simulink model "modelo"  (R2013a)
settings: Solver=ode45  StartTime=0.0  StopTime=50  FixedStep=0.01  RelTol=1e-3
values from neighbouring files (symbols this model uses):
  Hmax = [10 12 11 9]    [ini.m]
  Itot = [Ixx Ixy Izx; Ixy Iyy Iyz; Izx Iyz Izz]    [ini.m]
  Itot_inv = inv(Itot)    [ini.m]
  Iws = [5 5 5 5]    [ini.m]
  omega0 = [2000 2000 2000 2000]*rpm2r    [ini.m]
  r2d = 180/pi    (= 57.2957795131)    [ini.m]
  tau = [10;0;0]    [ini.m]
  w0 = [0.2 0.15 -0.18]*(pi/180.0)    [ini.m]
  w1 = [-1 -1 -1]/sqrt(3)    [ini.m]
  w2 = [-1 -1 +1]/sqrt(3)    [ini.m]
  w3 = [-1 +1 +1]/sqrt(3)    [ini.m]
  w4 = [-1 +1 -1]/sqrt(3)    [ini.m]
settings Model: Creator=henry  LastModifiedBy=henry
settings DataIOCC: InspectSignalLogs=on

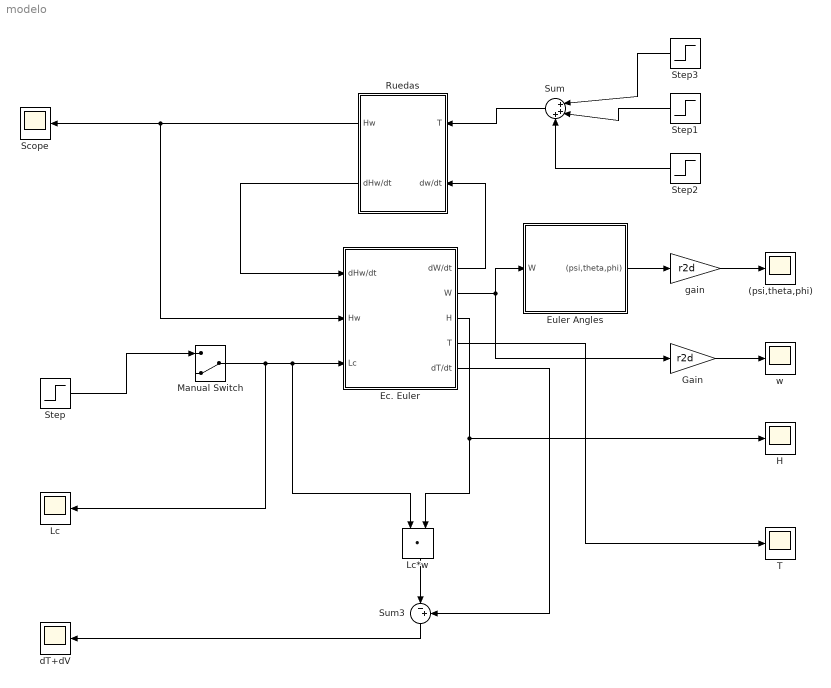
== system modelo ==
  (psi,theta,phi) : Scope
      settings: TickLabels=on  ShowLegends=on
  Ec. Euler : Subsystem
  Euler Angles : Subsystem
  Gain : Gain  Gain=r2d
  H : Scope
      settings: ShowLegends=on  SaveName=ScopeData4
  Lc : Scope
      settings: TickLabels=on  ShowLegends=on  SaveName=ScopeData2
  Lc*w : DotProduct  InputSameDT=on  OutDataTypeStr=Inherit: Inherit via internal rule
  Manual Switch : ManualSwitch  CurrentSetting=0
  Ruedas : Subsystem
  Scope : Scope
      settings: ShowLegends=on  SaveName=ScopeData9
  Step : Step  Time=1000  Before=[0;0;0]  After=tau  SampleTime=0
  Step1 : Step  Time=0  Before=[0;0;0]  After=tau  SampleTime=0
  Step2 : Step  Time=10  Before=[0;0;0]  After=-2*tau  SampleTime=0
  Step3 : Step  Time=15  Before=[0;0;0]  After=tau  SampleTime=0
  Sum : Sum  Inputs=|+++
  Sum3 : Sum  Inputs=|-+
  T : Scope
      settings: SaveName=ScopeData6
  dT+dV : Scope
      settings: TickLabels=on  ShowLegends=on  SaveName=ScopeData5
  gain : Gain  Gain=r2d
  w : Scope
      settings: TickLabels=on  ShowLegends=on
  wires:
  Lc*w/1 -> Sum3/1
  Sum3/1 -> dT+dV/1
  Ec. Euler/4(T) -> T/1
  Ec. Euler/5(dT/dt) -> Sum3/2
  Euler Angles/1((psi,theta,phi)) -> gain/1
  Gain/1 -> w/1
  gain/1 -> (psi,theta,phi)/1
  Ec. Euler/3(H) -> Lc*w/2, H/1
  Ec. Euler/2(W) -> Gain/1, Euler Angles/1(W)
  Ec. Euler/1(dW/dt) -> Ruedas/2(dw/dt)
  Ruedas/1(Hw) -> Ec. Euler/2(Hw), Scope/1
  Ruedas/2(dHw/dt) -> Ec. Euler/1(dHw/dt)
  Step1/1 -> Sum/2
  Step/1 -> Manual Switch/1
  Manual Switch/1 -> Lc/1, Lc*w/1, Ec. Euler/3(Lc)
  Step2/1 -> Sum/3
  Sum/1 -> Ruedas/1(T)
  Step3/1 -> Sum/1

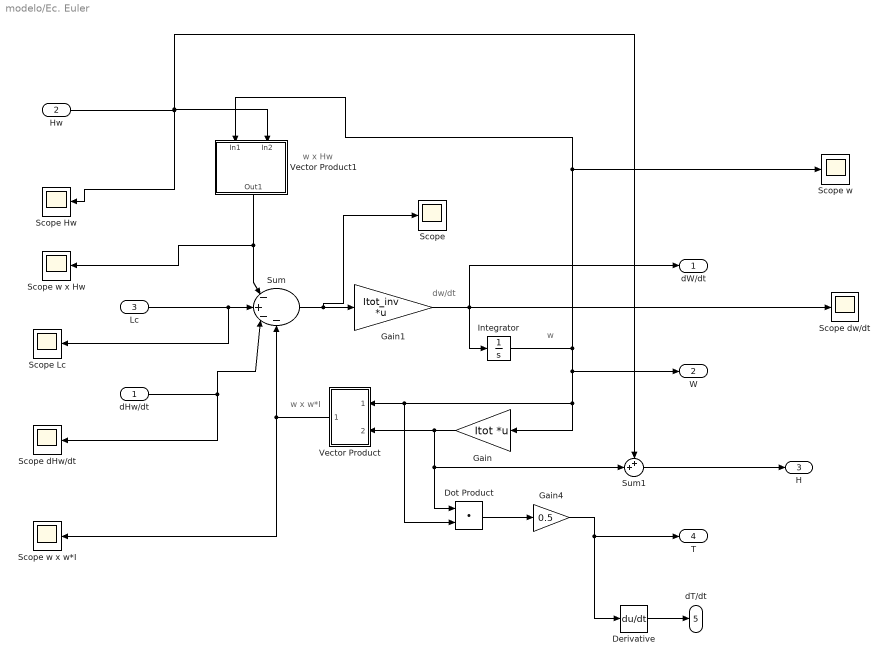
== system modelo/Ec. Euler ==
  note: w x w*I
  note: w x Hw
  note: w
  note: dw/dt
  dHw/dt : Inport
  Hw : Inport  Port=2
  Lc : Inport  Port=3
  Derivative : Derivative
  Dot Product : DotProduct  InputSameDT=on  OutDataTypeStr=Inherit: Inherit via internal rule
  Gain : Gain  Gain=Itot  Multiplication=Matrix(K*u)
  Gain1 : Gain  Gain=Itot_inv  Multiplication=Matrix(K*u)
  Gain4 : Gain  Gain=0.5
  Integrator : Integrator  InitialCondition=w0
  Scope : Scope
      settings: SaveName=ScopeData11
  Scope Hw : Scope
      settings: SaveName=ScopeData17
  Scope Lc : Scope
      settings: SaveName=ScopeData13
  Scope dHw/dt : Scope
      settings: SaveName=ScopeData14
  Scope dw/dt : Scope
      settings: SaveName=ScopeData18
  Scope w : Scope
      settings: SaveName=ScopeData16
  Scope w x Hw : Scope
      settings: SaveName=ScopeData15
  Scope w x w*I : Scope
      settings: SaveName=ScopeData19
  Sum : Sum  Inputs=|-+--
  Sum1 : Sum  Inputs=++|
  Vector Product : Subsystem
  Vector Product1 : Subsystem
  dW/dt : Outport
  W : Outport  Port=2
  H : Outport  Port=3
  T : Outport  Port=4
  dT/dt : Outport  Port=5
  wires:
  Vector Product/1(Out1) -> Scope w x w*I/1, Sum/4
  Gain/1 -> Sum1/2, Dot Product/1, Vector Product/2(In2)
  Gain1/1 -> dW/dt/1, Scope dw/dt/1, Integrator/1
  Derivative/1 -> dT/dt/1
  Integrator/1 -> W/1, Dot Product/2, Vector Product/1(In1), Gain/1, Vector Product1/1(In1), Scope w/1
  Lc/1 -> Scope Lc/1, Sum/2
  Dot Product/1 -> Gain4/1
  Gain4/1 -> T/1, Derivative/1
  dHw/dt/1 -> Sum/3, Scope dHw/dt/1
  Vector Product1/1(Out1) -> Sum/1, Scope w x Hw/1
  Hw/1 -> Scope Hw/1, Vector Product1/2(In2), Sum1/1
  Sum/1 -> Scope/1, Gain1/1
  Sum1/1 -> H/1

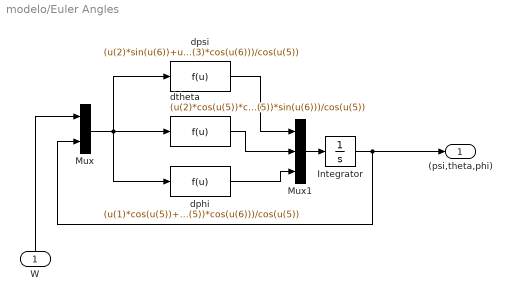
== system modelo/Euler Angles ==
  W : Inport
  Integrator : Integrator
  Mux : Mux  Inputs=2
  Mux1 : Mux  Inputs=3
  dphi : Fcn  Expr=(u(1)*cos(u(5))+u(2)*sin(u(5))*sin(u(6))+u(3)*sin(u(5))*cos(u(6)))/cos(u(5))
  dpsi : Fcn  Expr=(u(2)*sin(u(6))+u(3)*cos(u(6)))/cos(u(5))
  dtheta : Fcn  Expr=(u(2)*cos(u(5))*cos(u(6))-u(3)*cos(u(5))*sin(u(6)))/cos(u(5))
  (psi,theta,phi) : Outport
  wires:
  Integrator/1 -> (psi,theta,phi)/1, Mux/2
  dphi/1 -> Mux1/3
  dtheta/1 -> Mux1/2
  Mux1/1 -> Integrator/1
  dpsi/1 -> Mux1/1
  Mux/1 -> dpsi/1, dphi/1, dtheta/1
  W/1 -> Mux/1

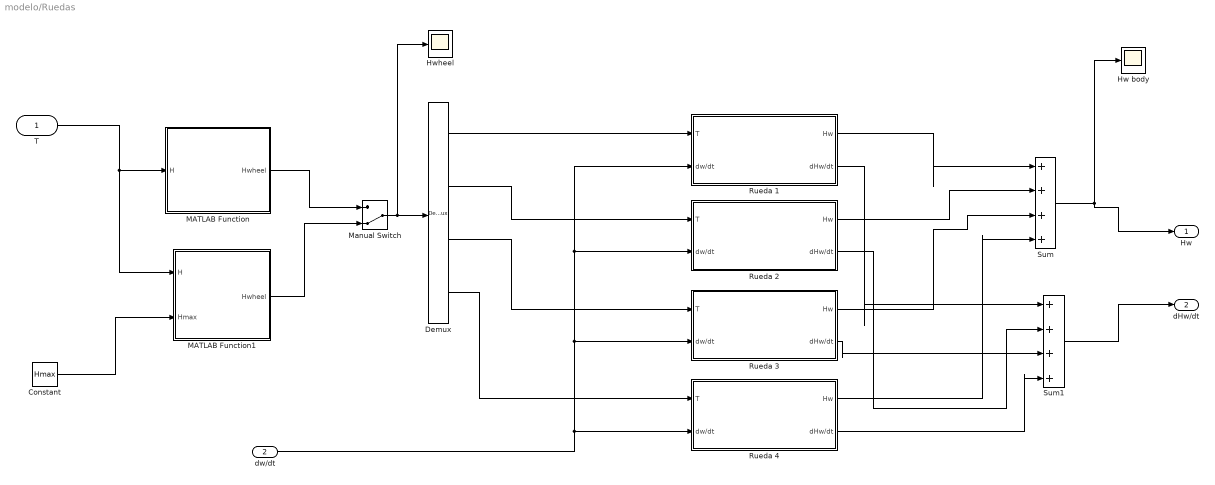
== system modelo/Ruedas ==
  T : Inport
  dw/dt : Inport  Port=2
  Constant : Constant  Value=Hmax
  Demux : Demux
  Hw body : Scope
      settings: ShowLegends=on  SaveName=ScopeData7
  Hwheel : Scope
      settings: ShowLegends=on  SaveName=ScopeData8
  MATLAB Function : MATLAB Function  TreatAsAtomicUnit=on
  MATLAB Function1 : MATLAB Function  TreatAsAtomicUnit=on
  Manual Switch : ManualSwitch  CurrentSetting=0
  Rueda 1 : Subsystem
  Rueda 2 : Subsystem
  Rueda 3 : Subsystem
  Rueda 4 : Subsystem
  Sum : Sum  Inputs=|++++
  Sum1 : Sum  Inputs=|++++
  Hw : Outport
  dHw/dt : Outport  Port=2
  wires:
  T/1 -> MATLAB Function1/1(H), MATLAB Function/1(H)
  Demux/1 -> Rueda 1/1(T)
  dw/dt/1 -> Rueda 2/2(dw/dt), Rueda 1/2(dw/dt), Rueda 3/2(dw/dt), Rueda 4/2(dw/dt)
  Demux/2 -> Rueda 2/1(T)
  Demux/3 -> Rueda 3/1(T)
  Demux/4 -> Rueda 4/1(T)
  Rueda 1/1(Hw) -> Sum/1
  Rueda 2/1(Hw) -> Sum/2
  Rueda 3/1(Hw) -> Sum/3
  Rueda 4/1(Hw) -> Sum/4
  Rueda 1/2(dHw/dt) -> Sum1/1
  Rueda 2/2(dHw/dt) -> Sum1/2
  Rueda 3/2(dHw/dt) -> Sum1/3
  Rueda 4/2(dHw/dt) -> Sum1/4
  Sum1/1 -> dHw/dt/1
  Sum/1 -> Hw/1, Hw body/1
  Constant/1 -> MATLAB Function1/2(Hmax)
  MATLAB Function1/1(Hwheel) -> Manual Switch/2
  MATLAB Function/1(Hwheel) -> Manual Switch/1
  Manual Switch/1 -> Hwheel/1, Demux/1

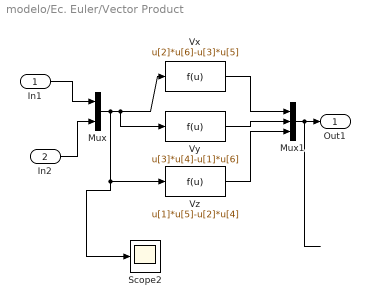
== system modelo/Ec. Euler/Vector Product ==
  In1 : Inport
  In2 : Inport  Port=2
  Mux : Mux  Inputs=2
  Mux1 : Mux  Inputs=3
  Scope2 : Scope
      settings: ShowLegends=on  SaveName=ScopeData3
  Vx : Fcn  Expr=u[2]*u[6]-u[3]*u[5]
  Vy : Fcn  Expr=u[3]*u[4]-u[1]*u[6]
  Vz : Fcn  Expr=u[1]*u[5]-u[2]*u[4]
  Out1 : Outport
  wires:
  In2/1 -> Mux/2
  Mux1/1 -> Out1/1
  In1/1 -> Mux/1
  Vz/1 -> Mux1/3
  Vy/1 -> Mux1/2
  Vx/1 -> Mux1/1
  Mux/1 -> Vz/1, Scope2/1, Vy/1, Vx/1

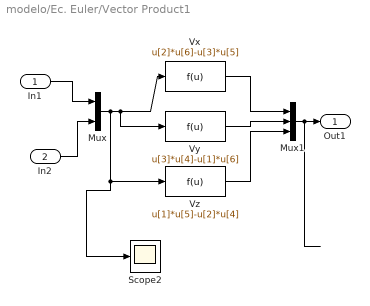
== system modelo/Ec. Euler/Vector Product1 ==
  In1 : Inport
  In2 : Inport  Port=2
  Mux : Mux  Inputs=2
  Mux1 : Mux  Inputs=3
  Scope2 : Scope
      settings: ShowLegends=on  SaveName=ScopeData3
  Vx : Fcn  Expr=u[2]*u[6]-u[3]*u[5]
  Vy : Fcn  Expr=u[3]*u[4]-u[1]*u[6]
  Vz : Fcn  Expr=u[1]*u[5]-u[2]*u[4]
  Out1 : Outport
  wires:
  In2/1 -> Mux/2
  Mux1/1 -> Out1/1
  In1/1 -> Mux/1
  Vz/1 -> Mux1/3
  Vy/1 -> Mux1/2
  Vx/1 -> Mux1/1
  Mux/1 -> Vz/1, Scope2/1, Vy/1, Vx/1

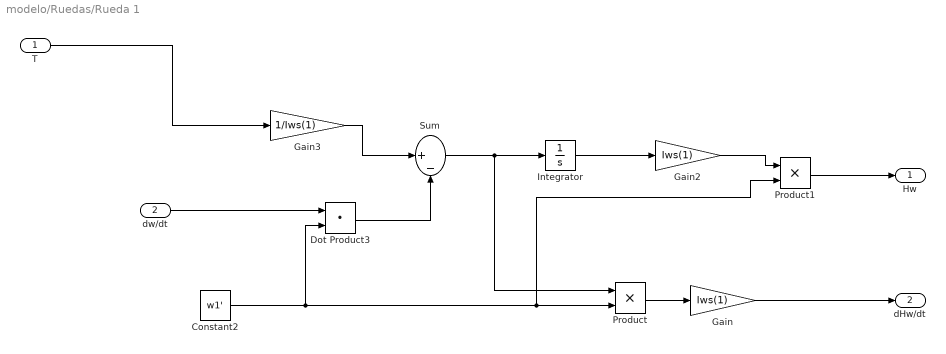
== system modelo/Ruedas/Rueda 1 ==
  T : Inport
  dw/dt : Inport  Port=2
  Constant2 : Constant  Value=w1'
  Dot Product3 : DotProduct  InputSameDT=on  OutDataTypeStr=Inherit: Inherit via internal rule
  Gain : Gain  Gain=Iws(1)
  Gain2 : Gain  Gain=Iws(1)
  Gain3 : Gain  Gain=1/Iws(1)
  Integrator : Integrator  InitialCondition=omega0(1)
  Product : Product
  Product1 : Product
  Sum : Sum  Inputs=|+-
  Hw : Outport
  dHw/dt : Outport  Port=2
  wires:
  Sum/1 -> Product/1, Integrator/1
  Gain3/1 -> Sum/1
  T/1 -> Gain3/1
  Dot Product3/1 -> Sum/2
  dw/dt/1 -> Dot Product3/1
  Integrator/1 -> Gain2/1
  Constant2/1 -> Product1/2, Product/2, Dot Product3/2
  Product/1 -> Gain/1
  Gain/1 -> dHw/dt/1
  Gain2/1 -> Product1/1
  Product1/1 -> Hw/1

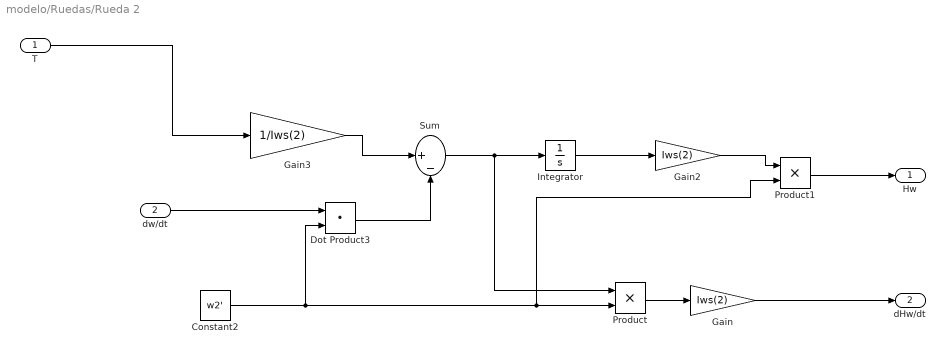
== system modelo/Ruedas/Rueda 2 ==
  T : Inport
  dw/dt : Inport  Port=2
  Constant2 : Constant  Value=w2'
  Dot Product3 : DotProduct  InputSameDT=on  OutDataTypeStr=Inherit: Inherit via internal rule
  Gain : Gain  Gain=Iws(2)
  Gain2 : Gain  Gain=Iws(2)
  Gain3 : Gain  Gain=1/Iws(2)
  Integrator : Integrator  InitialCondition=omega0(1)
  Product : Product
  Product1 : Product
  Sum : Sum  Inputs=|+-
  Hw : Outport
  dHw/dt : Outport  Port=2
  wires:
  Sum/1 -> Product/1, Integrator/1
  Gain3/1 -> Sum/1
  T/1 -> Gain3/1
  Dot Product3/1 -> Sum/2
  dw/dt/1 -> Dot Product3/1
  Integrator/1 -> Gain2/1
  Constant2/1 -> Product1/2, Product/2, Dot Product3/2
  Product/1 -> Gain/1
  Gain/1 -> dHw/dt/1
  Gain2/1 -> Product1/1
  Product1/1 -> Hw/1

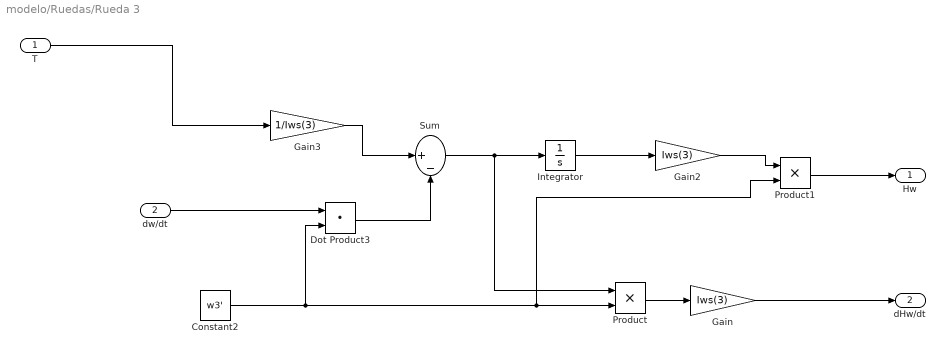
== system modelo/Ruedas/Rueda 3 ==
  T : Inport
  dw/dt : Inport  Port=2
  Constant2 : Constant  Value=w3'
  Dot Product3 : DotProduct  InputSameDT=on  OutDataTypeStr=Inherit: Inherit via internal rule
  Gain : Gain  Gain=Iws(3)
  Gain2 : Gain  Gain=Iws(3)
  Gain3 : Gain  Gain=1/Iws(3)
  Integrator : Integrator  InitialCondition=omega0(1)
  Product : Product
  Product1 : Product
  Sum : Sum  Inputs=|+-
  Hw : Outport
  dHw/dt : Outport  Port=2
  wires:
  Sum/1 -> Product/1, Integrator/1
  Gain3/1 -> Sum/1
  T/1 -> Gain3/1
  Dot Product3/1 -> Sum/2
  dw/dt/1 -> Dot Product3/1
  Integrator/1 -> Gain2/1
  Constant2/1 -> Product1/2, Product/2, Dot Product3/2
  Product/1 -> Gain/1
  Gain/1 -> dHw/dt/1
  Gain2/1 -> Product1/1
  Product1/1 -> Hw/1

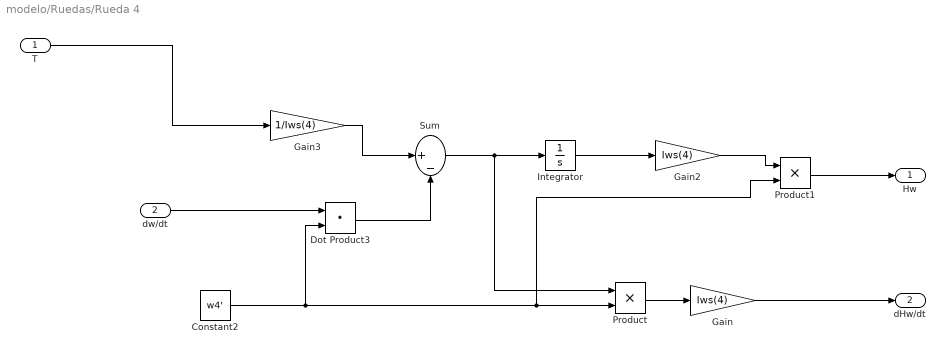
== system modelo/Ruedas/Rueda 4 ==
  T : Inport
  dw/dt : Inport  Port=2
  Constant2 : Constant  Value=w4'
  Dot Product3 : DotProduct  InputSameDT=on  OutDataTypeStr=Inherit: Inherit via internal rule
  Gain : Gain  Gain=Iws(4)
  Gain2 : Gain  Gain=Iws(4)
  Gain3 : Gain  Gain=1/Iws(4)
  Integrator : Integrator  InitialCondition=omega0(1)
  Product : Product
  Product1 : Product
  Sum : Sum  Inputs=|+-
  Hw : Outport
  dHw/dt : Outport  Port=2
  wires:
  Sum/1 -> Product/1, Integrator/1
  Gain3/1 -> Sum/1
  T/1 -> Gain3/1
  Dot Product3/1 -> Sum/2
  dw/dt/1 -> Dot Product3/1
  Integrator/1 -> Gain2/1
  Constant2/1 -> Product1/2, Product/2, Dot Product3/2
  Product/1 -> Gain/1
  Gain/1 -> dHw/dt/1
  Gain2/1 -> Product1/1
  Product1/1 -> Hw/1

== matlab function modelo/Ruedas/MATLAB Function1 ==
  data: H input; Hwheel output; Hmax input
function Hwheel  = ruedasLinfty_v02(H,Hmax)

% Orientacion de las ruedas y pre-calculos
w1 = [-1 -1 -1]/sqrt(3); % orientaciÃ³n de la rueda 1
w2 = [-1 -1 +1]/sqrt(3); % orientaciÃ³n de la rueda 2
w3 = [-1 +1 +1]/sqrt(3); % orientaciÃ³n de la rueda 3
w4 = [-1 +1 -1]/sqrt(3); % orientaciÃ³n de la rueda 4 
W = [w1' w2' w3' w4'];
[m n] = size(W);% numero de ruedas
% Calculo de las ruedas no saturadas k y l
N = zeros(n,n,3);
Hm = zeros(n,n);
facet = 0;
for i=1:n
    for j=1:n
        aux = cross(W(:,i),W(:,j));
        N(i,j,:) = aux;
        for m = 1:4
            Hm(i,j) = Hm(i,j)+Hmax(m)*abs(dot(W(:,m),aux));
        end
        if i~=j
            facet_aux = dot([N(i,j,1),N(i,j,2),N(i,j,3)],H)/Hm(i,j);
            if facet_aux <= facet
                facet = facet_aux;
                k = i;
                l = j;
            end
        end
    end
end

% Calculo en que sentido de giro se satura cada rueda
aux = 1:n; aux = aux(aux~=k); aux = aux(aux~=l);
aux2 = zeros(length(aux),1);
for i = 1: length(aux)
    aux2(i) = sign(dot(W(:,aux(i)),[N(k,l,1),N(k,l,2),N(k,l,3)]));
end
Hmax_aux = aux2.*Hmax(aux);

% Calculo de momento angular para cada rueda
M = [W(:,k) W(:,l) W(:,aux)*Hmax_aux];
sol = M\H;

% Construccion del vector HWheel
Hwheel = zeros(n,1);
Hwheel(k) = sol(1);
Hwheel(l) = sol(2);
for i=1:length(aux)
    Hwheel(aux(i))=sol(3)*Hmax_aux(i);
end

% % Verificacion
% if norm(H'-W*Hwheel)>1.0e-7
%     Hcalculado = W*Hwheel;
%     fprintf('Error al calcular HWheel\n');
%     fprintf('vector a calcular H = [%.3g,%0.3g,%0.3g]\n',H(1),H(2),H(3));
%     fprintf('vector calculado W*Hwheel = [%.3g,%0.3g,%0.3g]\n',Hcalculado(1),Hcalculado(2),Hcalculado(3));
% 
% else
% end

== matlab function modelo/Ruedas/MATLAB Function ==
  data: H input; Hwheel output
function Hwheel  = ruedasLinfty_v01(H)

% Orientacion de las ruedas y pre-calculos
% Estos datos tambien pueden ser parametros de entrada de la funcion.
w1 = [-1 -1 -1]/sqrt(3); % orientaciÃ³n de la rueda 1
w2 = [-1 -1 +1]/sqrt(3); % orientaciÃ³n de la rueda 2
w3 = [-1 +1 +1]/sqrt(3); % orientaciÃ³n de la rueda 3
w4 = [-1 +1 -1]/sqrt(3); % orientaciÃ³n de la rueda 4 
W = [w1' w2' w3' w4'];
[m n] = size(W);% numero de ruedas
N = zeros(n,n,3);
facet = 0;
for i=1:n
    for j=1:n
         N(i,j,:) = cross(W(:,i),W(:,j));
         if i~=j
            facet_aux = dot([N(i,j,1),N(i,j,2),N(i,j,3)],H);
            if facet_aux <= facet
                facet = facet_aux;
                k = i;
                l = j;
            end
         end
    end
end

% Calculo en que sentido de giro se satura cada rueda
aux = 1:n; aux = aux(aux~=k); aux = aux(aux~=l); % Esta sintaxis es la que marcha en Simulink
% aux = 1:n; aux([k,l])=[]; 
V = zeros(3,1); 
D = 0;
aux2 = zeros(length(aux),1);
for i =1: length(aux)
    aux2(i) = dot(W(:,aux(i)),[N(k,l,1),N(k,l,2),N(k,l,3)]);
    V(:) = V(:) + W(:,aux(i))*sign(aux2(i));
    D = D + norm(aux2(i));
end

% Calculo de momento angular para cada rueda
% M = [W(:,2) W(:,4) V];
% sol = M\H';
% HI = sol(1);
% HII = sol(2);
% H0 = sol(3);

% Solucion del sistema lineal de ecuaciones usando la regla de Crammer
aux_3 = dot(V,cross(W(:,k),W(:,l)))^-1;
HI = aux_3*(dot(cross(W(:,l),V),H)); % Momento angular rueda k no saturada
HII = aux_3*(dot(cross(V,W(:,k)),H)); % Momento angular rueda l no saturada
H0 = dot([N(k,l,1),N(k,l,2),N(k,l,3)],H)/D; %Momento angular ruedas saturadas

% Construccion del vector HWheel
Hwheel = zeros(4,1);
Hwheel(aux) = H0*sign(aux2);
Hwheel(k) = HI;
Hwheel(l) = HII;

% % Verificacion
% if norm(H'-W*Hwheel)>1.0e-7
%     Hcalculado = W*Hwheel;
%     fprintf('Error al calcular HWheel\n');
%     fprintf('vector a calcular H = [%.3g,%0.3g,%0.3g]\n',H(1),H(2),H(3));
%     fprintf('vector calculado W*Hwheel = [%.3g,%0.3g,%0.3g]\n',Hcalculado(1),Hcalculado(2),Hcalculado(3));
% else
end
